simulink model "wlanhdlTimeAndFrequencySynchronization"  (R2025a)
settings: Solver=FixedStepDiscrete  StartTime=0.0  StopTime=stopTime  RelTol=1e-3
InitFcn:
  | wlanFrontEndInit;
values from neighbouring files (symbols this model uses):
  filterLatency = (wlanConfig.corrLen/filterUpsampleFactor)+filterUpsampleFactor+9    [wlanFrontEndInit.m]
  filterUpsampleFactor = 160e6/wlanConfig.Fs    [wlanFrontEndInit.m]
  Hd = dfilt.dffir(b)    [wlanFrontEndInit.m]
undefined symbols (not defined in the file or in its folder): Add, Shift, wlanConfig
libraries: simulink x14, hdlsllib x9, dspsrcs4 x3, dspsigops x3, dsphdlsigops2 x2, dsphdlmathfun2 x2, dsphdlfiltering2 x2
(part 1 of 2)
settings Model: DataTypeOverride=Off  Creator=The MathWorks, Inc.  LastModifiedBy=The MathWorks, Inc.
settings SolverCC: MaxZcPerStep=1.0
settings OptimizationCC: BlockReduction=off  ConditionallyExecuteInputs=off  DefaultParameterBehavior=Inlined  ReuseModelBlockBuffer=off
settings DebuggingCC: AlgebraicLoopMsg=error  SaveWithParameterizedLinksMsg=none  SingleTaskRateTransMsg=error  UnconnectedInputMsg=warning  UnconnectedOutputMsg=warning  UnconnectedLineMsg=warning
settings HardwareCC: ProdBitPerPointer=32.0  ProdBitPerSizeT=32.0  ProdBitPerPtrDiffT=32.0  ProdLargestAtomicFloat=None  ProdIntDivRoundTo=Undefined  ProdEndianess=Unspecified  ProdWordSize=32.0  ProdHWDeviceType=ASIC/FPGA->ASIC/FPGA  TargetBitPerPointer=64.0  TargetBitPerSizeT=64.0  TargetBitPerPtrDiffT=64.0  TargetLongLongMode=on  TargetIntDivRoundTo=Zero  TargetEndianess=LittleEndian  TargetWordSize=64.0  TargetHWDeviceType=Custom Processor->MATLAB Host Computer  ProdEqTarget=off
settings ModelReferenceCC: EnableRefExpFcnMdlSchedulingChecks=on
settings RTWCC: GPUComputeCapability=3.5  DLArmComputeVersion=19.05

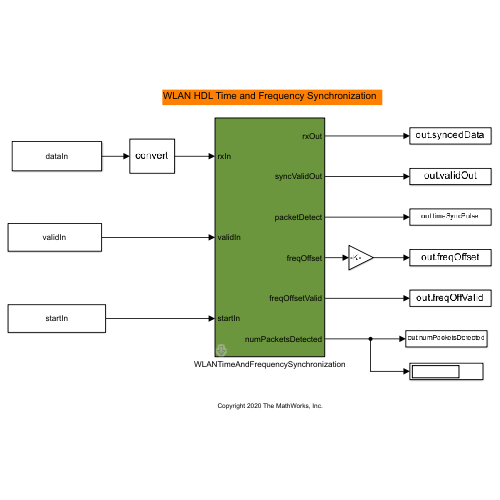
[thumbnail: Simulink's stored preview of the top-level diagram]
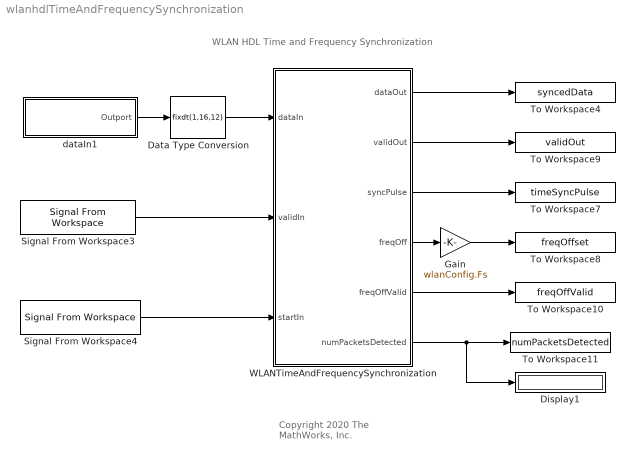
== system wlanhdlTimeAndFrequencySynchronization ==
  note: Copyright 2020 The MathWorks, Inc.
  note: WLAN HDL Time and Frequency Synchronization
  Data Type Conversion : DataTypeConversion  OutDataTypeStr=fixdt(1,16,12)  SaturateOnIntegerOverflow=off  RndMeth=Floor
  Display1 : Display
  Gain : Gain  Gain=wlanConfig.Fs
  Signal From Workspace3 : dspsrcs4/Signal From Workspace  X=validIn  Ts=1/wlanConfig.Fs  nsamps=1  OutputAfterFinalValue=Setting to zero  ignoreOrWarnInputAndFrameLengths=off  OutputFrames=off
  Signal From Workspace4 : dspsrcs4/Signal From Workspace  X=startIn  Ts=1/wlanConfig.Fs  nsamps=1  OutputAfterFinalValue=Setting to zero  ignoreOrWarnInputAndFrameLengths=off  OutputFrames=off
  To Workspace10 : ToWorkspace  VariableName=freqOffValid  SampleTime=-1
      settings: Save2DSignal=2-D array (concatenate along first dimension)
  To Workspace11 : ToWorkspace  VariableName=numPacketsDetected  SampleTime=-1
      settings: Save2DSignal=2-D array (concatenate along first dimension)
  To Workspace4 : ToWorkspace  VariableName=syncedData  SampleTime=-1
      settings: Save2DSignal=2-D array (concatenate along first dimension)
  To Workspace7 : ToWorkspace  VariableName=timeSyncPulse  SampleTime=-1
      settings: Save2DSignal=2-D array (concatenate along first dimension)
  To Workspace8 : ToWorkspace  VariableName=freqOffset  SampleTime=-1
      settings: Save2DSignal=2-D array (concatenate along first dimension)
  To Workspace9 : ToWorkspace  VariableName=validOut  SampleTime=-1
      settings: Save2DSignal=2-D array (concatenate along first dimension)
  WLANTimeAndFrequencySynchronization : Subsystem  mask(WLAN Front end application){chanBW=20MHz}
      mask prompts: chanBW "Channel bandwidth:"
      mask help: Performs time and frequency synchronization.
      mask Help: eval('showExample(''whdl/WLANHDLTimeAndFrequencySynchronizationExample'')')
      mask TypeOptions chanBW: 20MHz | 40MHz | 80MHz
      mask DialogControl DescGroupVar Prompt: WLAN Time and Frequency Synchronization
      mask DialogControl DescTextVar Prompt: Perform time and frequency synchronization.
      mask DialogControl ParameterGroupVar Prompt: Main
      mask Display:
      | port_label('input',1,'rxIn');
      | port_label('input',2,'validIn');
      | port_label('input',3,'startIn');
      | port_label('output',1,'rxOut');
      | port_label('output',2,'syncValidOut');
      | port_label('output',3,'packetDetect');
      | port_label('output',4,'freqOffset');
      | port_label('output',5,'freqOffsetValid');
      | 
      | port_label('output',6,'numPacketsDetected');
  dataIn1 : Subsystem
      mask Display: disp('dataIn');
  wires:
  Signal From Workspace3/1 -> WLANTimeAndFrequencySynchronization/2(validIn)
  WLANTimeAndFrequencySynchronization/5(freqOffValid) -> To Workspace10/1
  WLANTimeAndFrequencySynchronization/6(numPacketsDetected) -> To Workspace11/1, Display1/1
  WLANTimeAndFrequencySynchronization/3(syncPulse) -> To Workspace7/1
  Signal From Workspace4/1 -> WLANTimeAndFrequencySynchronization/3(startIn)
  WLANTimeAndFrequencySynchronization/2(validOut) -> To Workspace9/1
  WLANTimeAndFrequencySynchronization/1(dataOut) -> To Workspace4/1
  Data Type Conversion/1 -> WLANTimeAndFrequencySynchronization/1(dataIn)
  dataIn1/1(Outport) -> Data Type Conversion/1
  WLANTimeAndFrequencySynchronization/4(freqOff) -> Gain/1
  Gain/1 -> To Workspace8/1

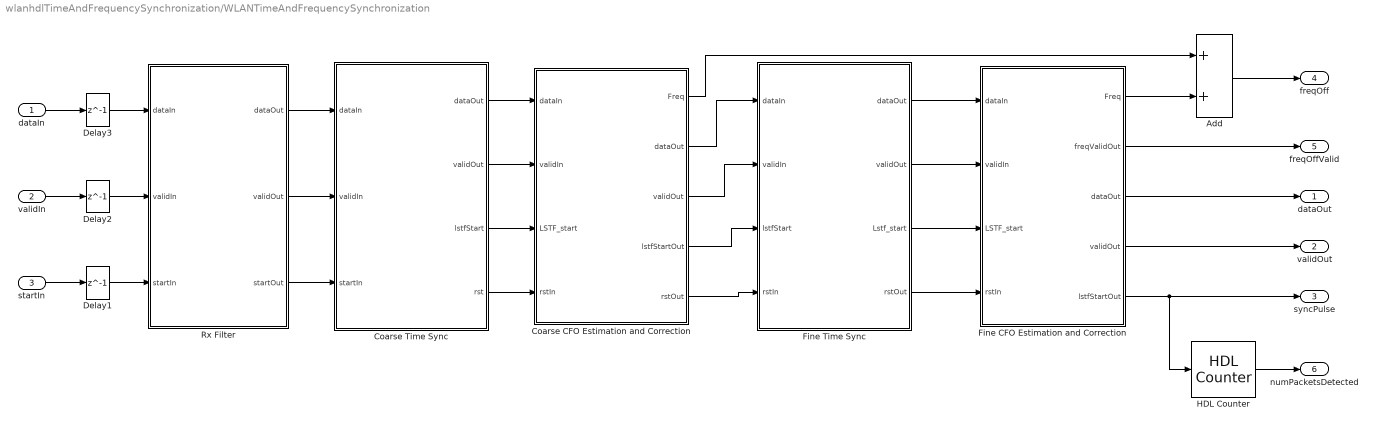
== system wlanhdlTimeAndFrequencySynchronization/WLANTimeAndFrequencySynchronization ==
  dataIn : Inport
  validIn : Inport  Port=2
  startIn : Inport  Port=3
  Add : Sum
  Coarse CFO Estimation and Correction : Subsystem
  Coarse Time Sync : Subsystem
  Delay1 : Delay  DelayLength=1  InitialCondition=0
  Delay2 : Delay  DelayLength=1  InitialCondition=0
  Delay3 : Delay  DelayLength=1  InitialCondition=0
  Fine CFO Estimation and Correction : Subsystem
  Fine Time Sync : Subsystem
  HDL Counter : hdlsllib/Sources/HDL Counter  CountType=Count limited  CountInit=0  CountStep=1  CountMax=65535  CountFromType=Initial value  CountFrom=0  CountResetPort=off  CountLoadPort=off  CountEnbPort=on  CountDirPort=off  CountHitOutputPort=off  CountDataType=Unsigned  CountWordLen=16  CountFracLen=0  CountSampTime=1
      link override Add_wrap/Compare To Constant/Compare: Operator=>  OutDataTypeStr=boolean
      link override Sub_wrap/Compare To Constant/Compare: Operator=<  OutDataTypeStr=boolean
      link override const_load_val: OutDataTypeStr=fixdt(issigned,CountWordLen,CountFracLen,'DataTypeOverride','Off')
  Rx Filter : Subsystem
  dataOut : Outport
  validOut : Outport  Port=2
  syncPulse : Outport  Port=3
  freqOff : Outport  Port=4
  freqOffValid : Outport  Port=5
  numPacketsDetected : Outport  Port=6
  wires:
  Add/1 -> freqOff/1
  validIn/1 -> Delay2/1
  dataIn/1 -> Delay3/1
  startIn/1 -> Delay1/1
  Delay1/1 -> Rx Filter/3(startIn)
  Rx Filter/3(startOut) -> Coarse Time Sync/3(startIn)
  Fine CFO Estimation and Correction/2(freqValidOut) -> freqOffValid/1
  HDL Counter/1 -> numPacketsDetected/1
  Delay3/1 -> Rx Filter/1(dataIn)
  Delay2/1 -> Rx Filter/2(validIn)
  Rx Filter/1(dataOut) -> Coarse Time Sync/1(dataIn)
  Rx Filter/2(validOut) -> Coarse Time Sync/2(validIn)
  Coarse Time Sync/1(dataOut) -> Coarse CFO Estimation and Correction/1(dataIn)
  Coarse Time Sync/2(validOut) -> Coarse CFO Estimation and Correction/2(validIn)
  Coarse Time Sync/3(lstfStart) -> Coarse CFO Estimation and Correction/3(LSTF_start)
  Coarse Time Sync/4(rst) -> Coarse CFO Estimation and Correction/4(rstIn)
  Coarse CFO Estimation and Correction/1(Freq) -> Add/1
  Coarse CFO Estimation and Correction/2(dataOut) -> Fine Time Sync/1(dataIn)
  Coarse CFO Estimation and Correction/3(validOut) -> Fine Time Sync/2(validIn)
  Coarse CFO Estimation and Correction/4(lstfStartOut) -> Fine Time Sync/3(lstfStart)
  Coarse CFO Estimation and Correction/5(rstOut) -> Fine Time Sync/4(rstIn)
  Fine CFO Estimation and Correction/5(lstfStartOut) -> syncPulse/1, HDL Counter/1
  Fine Time Sync/1(dataOut) -> Fine CFO Estimation and Correction/1(dataIn)
  Fine Time Sync/2(validOut) -> Fine CFO Estimation and Correction/2(validIn)
  Fine Time Sync/3(Lstf_start) -> Fine CFO Estimation and Correction/3(LSTF_start)
  Fine Time Sync/4(rstOut) -> Fine CFO Estimation and Correction/4(rstIn)
  Fine CFO Estimation and Correction/1(Freq) -> Add/2
  Fine CFO Estimation and Correction/3(dataOut) -> dataOut/1
  Fine CFO Estimation and Correction/4(validOut) -> validOut/1

== system wlanhdlTimeAndFrequencySynchronization/dataIn1 ==
  Signal From Workspace : dspsrcs4/Signal From Workspace  X=inputWaveform  Ts=1/wlanConfig.Fs  nsamps=1  OutputAfterFinalValue=Setting to zero  ignoreOrWarnInputAndFrameLengths=off  OutputFrames=off
  Outport : Outport
  wires:
  Signal From Workspace/1 -> Outport/1

== system wlanhdlTimeAndFrequencySynchronization/WLANTimeAndFrequencySynchronization/Coarse CFO Estimation and Correction ==
  dataIn : Inport
  validIn : Inport  Port=2
  LSTF_start : Inport  Port=3
  rstIn : Inport  Port=4
  Coarse CFO Correction : Subsystem
  Coarse CFO Estimation : Subsystem
  Freq : Outport
  dataOut : Outport  Port=2
  validOut : Outport  Port=3
  lstfStartOut : Outport  Port=4
  rstOut : Outport  Port=5
  wires:
  Coarse CFO Estimation/3(validData) -> Coarse CFO Correction/3(validIn)
  Coarse CFO Correction/3(validOut) -> validOut/1
  Coarse CFO Estimation/4(lstfStart) -> Coarse CFO Correction/4(lstfStartIn)
  Coarse CFO Estimation/1(Freq) -> Coarse CFO Correction/1(freq)
  LSTF_start/1 -> Coarse CFO Estimation/3(LSTF_start)
  validIn/1 -> Coarse CFO Estimation/2(validIn)
  Coarse CFO Estimation/5(rstOut) -> Coarse CFO Correction/5(rstIn)
  Coarse CFO Estimation/2(dataOut) -> Coarse CFO Correction/2(dataIn)
  dataIn/1 -> Coarse CFO Estimation/1(dataIn)
  Coarse CFO Correction/2(dataOut) -> dataOut/1
  rstIn/1 -> Coarse CFO Estimation/4(rstIn)
  Coarse CFO Correction/4(lstfStartOut) -> lstfStartOut/1
  Coarse CFO Correction/5(rstOut) -> rstOut/1
  Coarse CFO Correction/1(freqOut) -> Freq/1

== system wlanhdlTimeAndFrequencySynchronization/WLANTimeAndFrequencySynchronization/Coarse Time Sync ==
  dataIn : Inport
  validIn : Inport  Port=2
  startIn : Inport  Port=3
  Correlator : Subsystem
  Delay4 : Delay  DelayLength=7
  Delay6 : Delay  DelayLength=7
  Energy Calculator : Subsystem
  Peak Detector : Subsystem
  Stream Synchronizer : Subsystem
  dataOut : Outport  VectorParamsAs1DForOutWhenUnconnected=off
  validOut : Outport  Port=2  VectorParamsAs1DForOutWhenUnconnected=off
  lstfStart : Outport  Port=3  VectorParamsAs1DForOutWhenUnconnected=off
  rst : Outport  Port=4  VectorParamsAs1DForOutWhenUnconnected=off
  wires:
  startIn/1 -> rst/1, Correlator/3(startIn)
  Peak Detector/3(dataOut) -> dataOut/1
  validIn/1 -> Delay6/1, Correlator/2(validIn), Energy Calculator/4(validIn)
  Delay4/1 -> Stream Synchronizer/2(dataIn)
  Delay6/1 -> Stream Synchronizer/3(dataValid)
  Correlator/2(validOut) -> Energy Calculator/2(corrValidIn), Stream Synchronizer/1(corrValid)
  dataIn/1 -> Energy Calculator/3(dataIn), Delay4/1, Correlator/1(dataIn)
  Peak Detector/2(validOut) -> validOut/1
  Energy Calculator/2(energyOut) -> Peak Detector/2(energyIn)
  Energy Calculator/3(validOut) -> Peak Detector/3(corrValid)
  Peak Detector/1(lstfStart) -> lstfStart/1
  Correlator/1(dataOut) -> Energy Calculator/1(corrIn)
  Energy Calculator/1(corrOut) -> Peak Detector/1(corrIn)
  Stream Synchronizer/1(dataOut) -> Peak Detector/4(dataIn)
  Stream Synchronizer/2(validOut) -> Peak Detector/5(dataValid)

== system wlanhdlTimeAndFrequencySynchronization/WLANTimeAndFrequencySynchronization/Fine CFO Estimation and Correction ==
  dataIn : Inport
  validIn : Inport  Port=2
  LSTF_start : Inport  Port=3
  rstIn : Inport  Port=4
  Fine CFO Correction : Subsystem
  Fine CFO Estimation : Subsystem
  Freq : Outport
  freqValidOut : Outport  Port=2
  dataOut : Outport  Port=3
  validOut : Outport  Port=4
  lstfStartOut : Outport  Port=5
  wires:
  Fine CFO Estimation/4(validOut) -> Fine CFO Correction/4(validIn)
  Fine CFO Estimation/1(Freq) -> Fine CFO Correction/1(freqIn)
  validIn/1 -> Fine CFO Estimation/2(validIn)
  Fine CFO Estimation/5(lstfStart) -> Fine CFO Correction/5(lstfStartIn)
  Fine CFO Estimation/3(dataOut) -> Fine CFO Correction/3(dataIn)
  dataIn/1 -> Fine CFO Estimation/1(dataIn)
  Fine CFO Estimation/2(freqValidOut) -> Fine CFO Correction/2(freqValidIn)
  LSTF_start/1 -> Fine CFO Estimation/3(LSTF_start)
  rstIn/1 -> Fine CFO Estimation/4(rstIn)
  Fine CFO Correction/5(lstfStartOut) -> lstfStartOut/1
  Fine CFO Correction/4(validOut) -> validOut/1
  Fine CFO Correction/3(dataOut) -> dataOut/1
  Fine CFO Correction/1(freqOut) -> Freq/1
  Fine CFO Correction/2(freqValidOut) -> freqValidOut/1

== system wlanhdlTimeAndFrequencySynchronization/WLANTimeAndFrequencySynchronization/Fine Time Sync ==
  dataIn : Inport
  validIn : Inport  Port=2
  lstfStart : Inport  Port=3
  rstIn : Inport  Port=4
  Correlator : Subsystem
  Peak Searcher : Subsystem
  dataOut : Outport  VectorParamsAs1DForOutWhenUnconnected=off
  validOut : Outport  Port=2  VectorParamsAs1DForOutWhenUnconnected=off
  Lstf_start : Outport  Port=3  VectorParamsAs1DForOutWhenUnconnected=off
  rstOut : Outport  Port=4  VectorParamsAs1DForOutWhenUnconnected=off
  wires:
  validIn/1 -> Correlator/2(validIn)
  dataIn/1 -> Correlator/1(dataIn)
  lstfStart/1 -> Correlator/3(startIn)
  Correlator/1(corrOut) -> Peak Searcher/1(corrIn)
  Correlator/2(corrValid) -> Peak Searcher/2(corrValid)
  Correlator/3(startOut) -> Peak Searcher/3(startIn)
  Peak Searcher/1(lstfStart) -> Lstf_start/1
  Peak Searcher/2(validOut) -> validOut/1
  Peak Searcher/3(dataOut) -> dataOut/1
  Correlator/4(dataOut) -> Peak Searcher/4(dataIn)
  Correlator/5(validOut) -> Peak Searcher/5(validIn)
  rstIn/1 -> rstOut/1, Peak Searcher/6(rstIn), Correlator/4(rstIn)

== system wlanhdlTimeAndFrequencySynchronization/WLANTimeAndFrequencySynchronization/Rx Filter ==
  dataIn : Inport
  validIn : Inport  Port=2
  startIn : Inport  Port=3
  DTConverter : MATLAB Function  TreatAsAtomicUnit=on
  Delay : Delay  DelayLength=33
  Discrete FIR Filter : dsphdlfiltering2/Discrete FIR Filter  NumeratorSource=Property  Numerator=Hd.Numerator  NumeratorPrototype=[]  FilterStructure=Direct form systolic  SerializationOption=Minimum number of cycles between valid input samples  NumCycles=2  NumberOfMultipliers=2  SimulateUsing=Code generation  roundingMode=Floor  overflowMode=off  CoefficientsDataTypeStr=Inherit: Same word length as input  OutputDataTypeStr=Inherit: Same word length as input  ResetInputPort=on  HDLGlobalReset=off  CoeffMultiplier=Multiplier  UseMultForPow2Coeff=on  FrameInputSymmOptim=off
  dataOut : Outport
  validOut : Outport  Port=2
  startOut : Outport  Port=3
  wires:
  dataIn/1 -> DTConverter/1(dataIn1), Discrete FIR Filter/1
  validIn/1 -> Discrete FIR Filter/2
  Discrete FIR Filter/2 -> validOut/1
  Discrete FIR Filter/1 -> DTConverter/2(dataIn2)
  DTConverter/1(dataOut) -> dataOut/1
  startIn/1 -> Discrete FIR Filter/3, Delay/1
  Delay/1 -> startOut/1

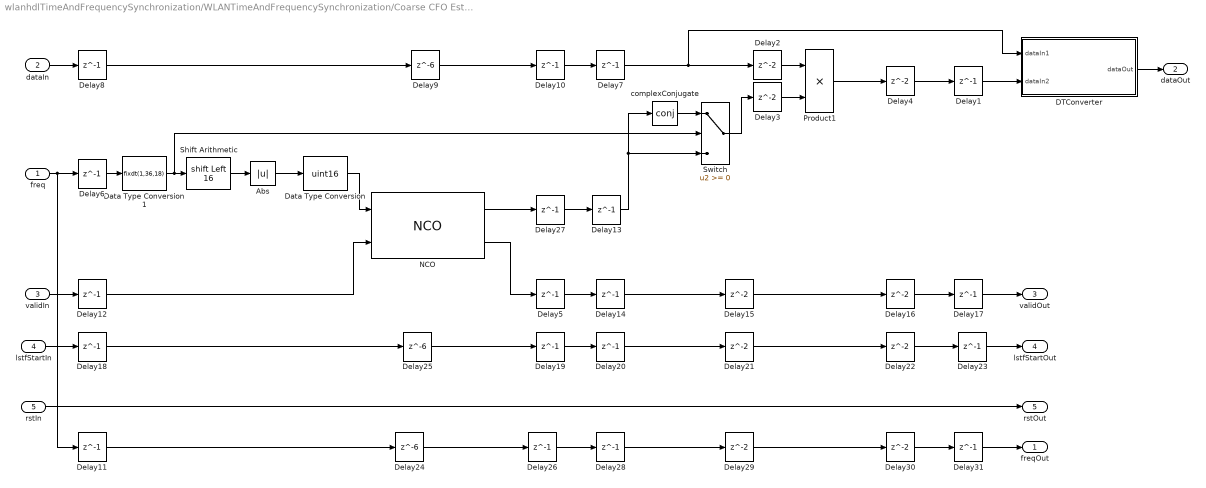
== system wlanhdlTimeAndFrequencySynchronization/WLANTimeAndFrequencySynchronization/Coarse CFO Estimation and Correction/Coarse CFO Correction ==
  freq : Inport
  dataIn : Inport  Port=2
  validIn : Inport  Port=3
  lstfStartIn : Inport  Port=4
  rstIn : Inport  Port=5
  Abs : Abs  SaturateOnIntegerOverflow=off
  DTConverter : MATLAB Function  TreatAsAtomicUnit=on
  Data Type Conversion : DataTypeConversion  OutDataTypeStr=uint16  RndMeth=Round  SaturateOnIntegerOverflow=off
  Data Type Conversion1 : DataTypeConversion  OutDataTypeStr=fixdt(1,36,18)  SaturateOnIntegerOverflow=off  RndMeth=Floor
  Delay{1,5..8,10..14,17..20,23,26..28,31} (19 alike) : Delay  DelayLength=1  InitialCondition=0  UseCircularBuffer=on
  Delay{2..4,15..16,21..22,29..30} (9 alike) : Delay  InitialCondition=0  UseCircularBuffer=on
  Delay24 : Delay  DelayLength=6  InitialCondition=0  UseCircularBuffer=on
  Delay25 : Delay  DelayLength=6  InitialCondition=0  UseCircularBuffer=on
  Delay9 : Delay  DelayLength=6  InitialCondition=0  UseCircularBuffer=on
  NCO : dsphdlsigops2/NCO  PhaseIncrementSource=Input port  PhaseIncrement=100  PhaseOffsetSource=Property  PhaseOffset=0  DitherSource=None  NumDitherBits=4  SamplesPerFrame=1  LUTCompress=off  ResetAction=off  Waveform=Complex exponential  PhasePort=off  SimulateUsing=Code generation  AccumulatorWL=16  PhaseQuantization=on  NumQuantizerAccumulatorBits=16  OutputDataType=Binary point scaling  OutputWL=16  OutputFL=14
  Product1 : Product
  Shift Arithmetic : ArithShift  BitShiftNumber=16  BitShiftDirection=Left
  Switch : Switch  SaturateOnIntegerOverflow=off  InputSameDT=off
  complexConjugate : Math  Operator=conj  SignedPower=on
  freqOut : Outport  VectorParamsAs1DForOutWhenUnconnected=off
  dataOut : Outport  Port=2  VectorParamsAs1DForOutWhenUnconnected=off
  validOut : Outport  Port=3  VectorParamsAs1DForOutWhenUnconnected=off
  lstfStartOut : Outport  Port=4  VectorParamsAs1DForOutWhenUnconnected=off
  rstOut : Outport  Port=5  VectorParamsAs1DForOutWhenUnconnected=off
  wires:
  Delay25/1 -> Delay19/1
  NCO/2 -> Delay5/1
  Delay9/1 -> Delay10/1
  Delay23/1 -> lstfStartOut/1
  Delay22/1 -> Delay23/1
  Delay21/1 -> Delay22/1
  Delay20/1 -> Delay21/1
  Delay19/1 -> Delay20/1
  Delay18/1 -> Delay25/1
  lstfStartIn/1 -> Delay18/1
  Delay5/1 -> Delay14/1
  freq/1 -> Delay11/1, Delay6/1
  Delay4/1 -> Delay1/1
  dataIn/1 -> Delay8/1
  Delay17/1 -> validOut/1
  Delay3/1 -> Product1/2
  Delay16/1 -> Delay17/1
  validIn/1 -> Delay12/1
  Delay10/1 -> Delay7/1
  Delay15/1 -> Delay16/1
  Delay2/1 -> Product1/1
  Product1/1 -> Delay4/1
  Delay13/1 -> complexConjugate/1, Switch/3
  Delay8/1 -> Delay9/1
  Delay7/1 -> DTConverter/1(dataIn1), Delay2/1
  Delay14/1 -> Delay15/1
  Delay27/1 -> Delay13/1
  Data Type Conversion/1 -> NCO/1
  Delay12/1 -> NCO/2
  NCO/1 -> Delay27/1
  rstIn/1 -> rstOut/1
  Delay6/1 -> Data Type Conversion1/1
  Data Type Conversion1/1 -> Switch/2, Shift Arithmetic/1
  DTConverter/1(dataOut) -> dataOut/1
  Delay1/1 -> DTConverter/2(dataIn2)
  complexConjugate/1 -> Switch/1
  Switch/1 -> Delay3/1
  Shift Arithmetic/1 -> Abs/1
  Abs/1 -> Data Type Conversion/1
  Delay11/1 -> Delay24/1
  Delay24/1 -> Delay26/1
  Delay26/1 -> Delay28/1
  Delay28/1 -> Delay29/1
  Delay29/1 -> Delay30/1
  Delay30/1 -> Delay31/1
  Delay31/1 -> freqOut/1

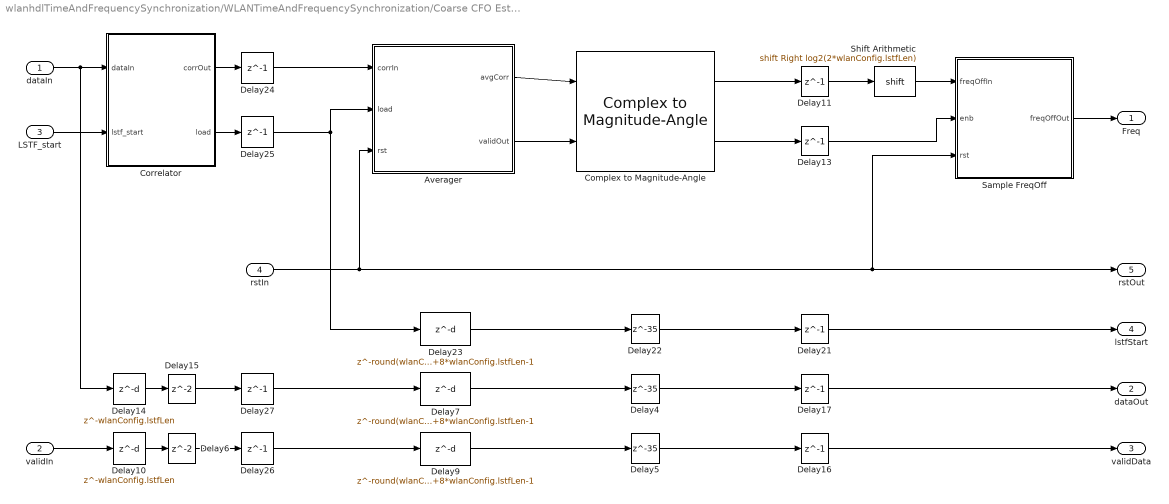
== system wlanhdlTimeAndFrequencySynchronization/WLANTimeAndFrequencySynchronization/Coarse CFO Estimation and Correction/Coarse CFO Estimation ==
  dataIn : Inport
  validIn : Inport  Port=2
  LSTF_start : Inport  Port=3
  rstIn : Inport  Port=4
  Averager : Subsystem
  Complex to Magnitude-Angle : dsphdlmathfun2/Complex to Magnitude-Angle  NumIterationsSource=Auto  NumIterations=30  OutputFormat=Angle  AngleFormat=Normalized  ScaleOutput=off  ScalingMethod=Shift-Add  SimulateUsing=Code generation
  Correlator : Subsystem
  Delay10 : Delay  DelayLength=wlanConfig.lstfLen  InitialCondition=0
  Delay{11,13,16..17,21} (5 alike) : Delay  DelayLength=1  InitialCondition=0  UseCircularBuffer=on
  Delay14 : Delay  DelayLength=wlanConfig.lstfLen  InitialCondition=0
  Delay15 : Delay  InitialCondition=0  UseCircularBuffer=on
  Delay22 : Delay  DelayLength=35  InitialCondition=0  UseCircularBuffer=on
  Delay23 : Delay  DelayLength=round(wlanConfig.lstfLen*0.75)+8*wlanConfig.lstfLen-1  InitialCondition=0  UseCircularBuffer=on
  Delay{24..27} (4 alike) : Delay  DelayLength=1
  Delay4 : Delay  DelayLength=35  InitialCondition=0  UseCircularBuffer=on
  Delay5 : Delay  DelayLength=35  InitialCondition=0  UseCircularBuffer=on
  Delay6 : Delay  InitialCondition=0  UseCircularBuffer=on
  Delay7 : Delay  DelayLength=round(wlanConfig.lstfLen*0.75)+8*wlanConfig.lstfLen-1  InitialCondition=0  UseCircularBuffer=on
  Delay9 : Delay  DelayLength=round(wlanConfig.lstfLen*0.75)+8*wlanConfig.lstfLen-1  InitialCondition=0  UseCircularBuffer=on
  Sample FreqOff : MATLAB Function  TreatAsAtomicUnit=on
  Shift Arithmetic : ArithShift  BitShiftNumber=log2(2*wlanConfig.lstfLen)  BitShiftDirection=Right
  Freq : Outport  VectorParamsAs1DForOutWhenUnconnected=off
  dataOut : Outport  Port=2  VectorParamsAs1DForOutWhenUnconnected=off
  validData : Outport  Port=3  VectorParamsAs1DForOutWhenUnconnected=off
  lstfStart : Outport  Port=4  VectorParamsAs1DForOutWhenUnconnected=off
  rstOut : Outport  Port=5  VectorParamsAs1DForOutWhenUnconnected=off
  wires:
  validIn/1 -> Delay10/1
  dataIn/1 -> Delay14/1, Correlator/1(dataIn)
  LSTF_start/1 -> Correlator/2(lstf_start)
  Delay9/1 -> Delay5/1
  Complex to Magnitude-Angle/2 -> Delay13/1
  Delay5/1 -> Delay16/1
  Delay4/1 -> Delay17/1
  Complex to Magnitude-Angle/1 -> Delay11/1
  Delay16/1 -> validData/1
  Delay17/1 -> dataOut/1
  Delay10/1 -> Delay6/1
  Delay6/1 -> Delay26/1
  Delay11/1 -> Shift Arithmetic/1
  Delay7/1 -> Delay4/1
  Delay26/1 -> Delay9/1
  Delay14/1 -> Delay15/1
  Delay15/1 -> Delay27/1
  Delay27/1 -> Delay7/1
  Delay22/1 -> Delay21/1
  Correlator/2(load) -> Delay25/1
  Delay23/1 -> Delay22/1
  Delay21/1 -> lstfStart/1
  Delay25/1 -> Delay23/1, Averager/2(load)
  Shift Arithmetic/1 -> Sample FreqOff/1(freqOffIn)
  Sample FreqOff/1(freqOffOut) -> Freq/1
  Delay13/1 -> Sample FreqOff/2(enb)
  rstIn/1 -> rstOut/1, Sample FreqOff/3(rst), Averager/3(rst)
  Correlator/1(corrOut) -> Delay24/1
  Averager/1(avgCorr) -> Complex to Magnitude-Angle/1
  Averager/2(validOut) -> Complex to Magnitude-Angle/2
  Delay24/1 -> Averager/1(corrIn)

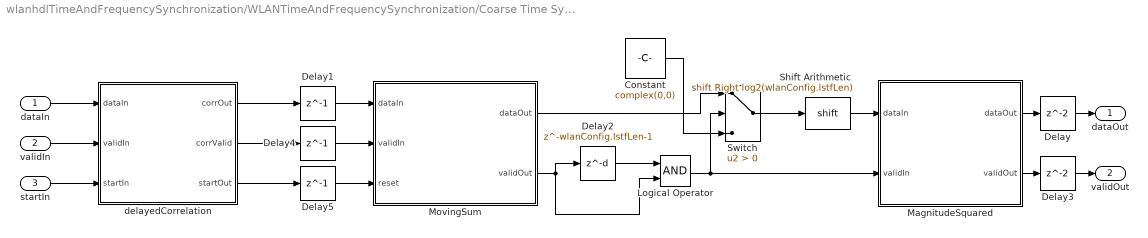
== system wlanhdlTimeAndFrequencySynchronization/WLANTimeAndFrequencySynchronization/Coarse Time Sync/Correlator ==
  dataIn : Inport
  validIn : Inport  Port=2
  startIn : Inport  Port=3
  Constant : Constant  Value=complex(0,0)  VectorParams1D=off  OutDataTypeStr=Inherit: Inherit via back propagation  SampleTime=-1
  Delay : Delay
  Delay1 : Delay  DelayLength=1
  Delay2 : Delay  DelayLength=wlanConfig.lstfLen-1
  Delay3 : Delay
  Delay4 : Delay  DelayLength=1
  Delay5 : Delay  DelayLength=1
  Logical Operator : Logic  AllPortsSameDT=off  OutDataTypeStr=boolean
  MagnitudeSquared : Subsystem
  MovingSum : Subsystem  InitFcn=Simulink.suppressDiagnostic(gcb, 'SimulinkFixedPoint:util:Overflowoccurred');
  Shift Arithmetic : ArithShift  BitShiftNumber=log2(wlanConfig.lstfLen)  BitShiftDirection=Right
  Switch : Switch  Criteria=u2 > Threshold  SaturateOnIntegerOverflow=off  InputSameDT=off
  delayedCorrelation : Subsystem
  dataOut : Outport
  validOut : Outport  Port=2
  wires:
  MagnitudeSquared/2(validOut) -> Delay3/1
  MovingSum/2(validOut) -> Delay2/1, Logical Operator/2
  Switch/1 -> Shift Arithmetic/1
  Constant/1 -> Switch/3
  MovingSum/1(dataOut) -> Switch/1
  Logical Operator/1 -> MagnitudeSquared/2(validIn), Switch/2
  Delay2/1 -> Logical Operator/1
  MagnitudeSquared/1(dataOut) -> Delay/1
  Shift Arithmetic/1 -> MagnitudeSquared/1(dataIn)
  Delay/1 -> dataOut/1
  Delay3/1 -> validOut/1
  dataIn/1 -> delayedCorrelation/1(dataIn)
  validIn/1 -> delayedCorrelation/2(validIn)
  startIn/1 -> delayedCorrelation/3(startIn)
  delayedCorrelation/1(corrOut) -> Delay1/1
  delayedCorrelation/2(corrValid) -> Delay4/1
  delayedCorrelation/3(startOut) -> Delay5/1
  Delay1/1 -> MovingSum/1(dataIn)
  Delay4/1 -> MovingSum/2(validIn)
  Delay5/1 -> MovingSum/3(reset)

== system wlanhdlTimeAndFrequencySynchronization/WLANTimeAndFrequencySynchronization/Coarse Time Sync/Energy Calculator ==
  corrIn : Inport
  corrValidIn : Inport  Port=2
  dataIn : Inport  Port=3
  validIn : Inport  Port=4
  Delay : Delay  DelayLength=3
  magnitudeSquared : Subsystem
  streamSynchronizer : Subsystem
  corrOut : Outport
  energyOut : Outport  Port=2
  validOut : Outport  Port=3
  wires:
  validIn/1 -> magnitudeSquared/2(validIn)
  streamSynchronizer/1(dataOut) -> energyOut/1
  magnitudeSquared/1(energy) -> streamSynchronizer/2(energy)
  corrValidIn/1 -> streamSynchronizer/1(corrValid)
  streamSynchronizer/2(validOut) -> validOut/1
  magnitudeSquared/2(push) -> streamSynchronizer/3(dataValid)
  dataIn/1 -> magnitudeSquared/1(dataIn)
  corrIn/1 -> Delay/1
  Delay/1 -> corrOut/1

== system wlanhdlTimeAndFrequencySynchronization/WLANTimeAndFrequencySynchronization/Coarse Time Sync/Peak Detector ==
  note: Searching peak in LSTF region
  corrIn : Inport
  energyIn : Inport  Port=2
  corrValid : Inport  Port=3
  dataIn : Inport  Port=4
  dataValid : Inport  Port=5
  Delay1 : Delay  DelayLength=wlanConfig.lstfLen*10  InitialCondition=0  UseCircularBuffer=on
  Delay2 : Delay  DelayLength=wlanConfig.lstfLen*10  InitialCondition=0  UseCircularBuffer=on
  Logical Operator3 : Logic  AllPortsSameDT=off  OutDataTypeStr=boolean
  MATLAB Function1 : MATLAB Function  TreatAsAtomicUnit=on
  Relational Operator : RelationalOperator  Operator=>  OutDataTypeStr=boolean  InputSameDT=off
  considerFirstPeak : Subsystem
  searchStartOfFrame : MATLAB Function  TreatAsAtomicUnit=on
  lstfStart : Outport
  validOut : Outport  Port=2
  dataOut : Outport  Port=3
  wires:
  Relational Operator/1 -> searchStartOfFrame/1(thresholdValid)
  Logical Operator3/1 -> validOut/1, MATLAB Function1/1(syncEn)
  energyIn/1 -> Relational Operator/2
  dataValid/1 -> Delay1/1
  corrValid/1 -> searchStartOfFrame/2(valid)
  dataIn/1 -> Delay2/1
  Delay2/1 -> MATLAB Function1/2(dataIn)
  Delay1/1 -> MATLAB Function1/3(validIn), Logical Operator3/2
  MATLAB Function1/1(dataOut) -> dataOut/1
  searchStartOfFrame/1(syncOut) -> considerFirstPeak/1(peakIn)
  considerFirstPeak/1(peakOut) -> lstfStart/1
  considerFirstPeak/2(validOut) -> Logical Operator3/1
  corrIn/1 -> Relational Operator/1

== system wlanhdlTimeAndFrequencySynchronization/WLANTimeAndFrequencySynchronization/Coarse Time Sync/Stream Synchronizer ==
  corrValid : Inport
  dataIn : Inport  Port=2
  dataValid : Inport  Port=3
  Delay{1..4,6} (5 alike) : Delay  DelayLength=1
  Delay5 : Delay  DelayLength=wlanConfig.lstfLen-1
  Logical Operator8 : Logic  Operator=OR  AllPortsSameDT=off  OutDataTypeStr=boolean
  StreamSyncronizer : MATLAB Function  InitFcn=Simulink.suppressDiagnostic(gcb, 'Stateflow:Runtime:DataOverflowErrorMSLD');  TreatAsAtomicUnit=on  mask{depth=256}
      mask help: Synchronize two data streams with a FIFO.
  dataOut : Outport
  validOut : Outport  Port=2
  wires:
  dataIn/1 -> Delay4/1
  Delay6/1 -> StreamSyncronizer/3(push)
  Delay4/1 -> StreamSyncronizer/2(dataIn)
  StreamSyncronizer/2(validOut) -> Delay3/1
  dataValid/1 -> Delay6/1
  StreamSyncronizer/1(dataOut) -> Delay2/1
  Delay1/1 -> StreamSyncronizer/1(pop)
  Delay2/1 -> dataOut/1
  Delay3/1 -> validOut/1
  corrValid/1 -> Logical Operator8/2, Delay5/1
  Delay5/1 -> Logical Operator8/1
  Logical Operator8/1 -> Delay1/1

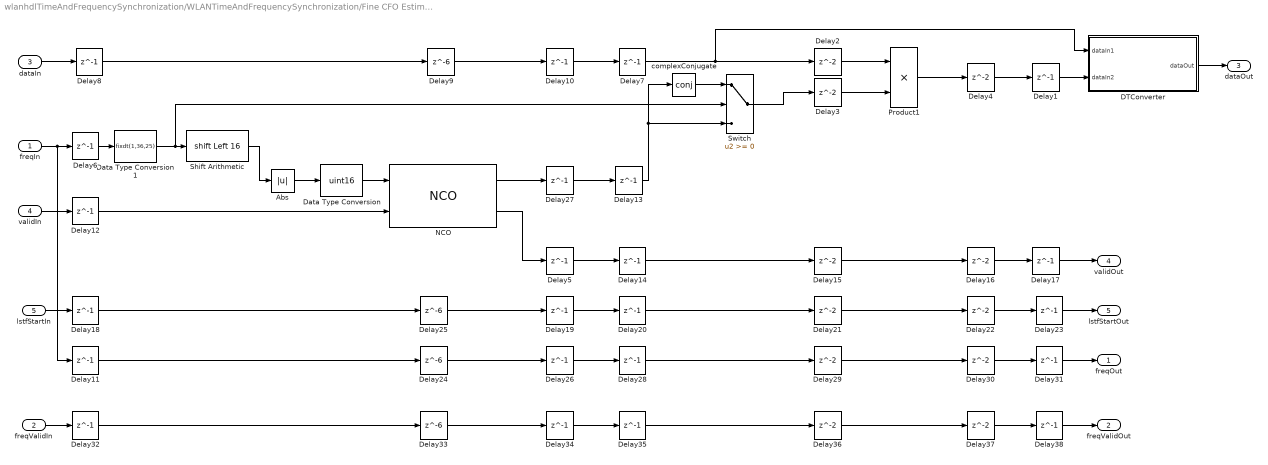
== system wlanhdlTimeAndFrequencySynchronization/WLANTimeAndFrequencySynchronization/Fine CFO Estimation and Correction/Fine CFO Correction ==
  freqIn : Inport
  freqValidIn : Inport  Port=2
  dataIn : Inport  Port=3
  validIn : Inport  Port=4
  lstfStartIn : Inport  Port=5
  Abs : Abs  SaturateOnIntegerOverflow=off
  DTConverter : MATLAB Function  TreatAsAtomicUnit=on
  Data Type Conversion : DataTypeConversion  OutDataTypeStr=uint16  RndMeth=Round  SaturateOnIntegerOverflow=off
  Data Type Conversion1 : DataTypeConversion  OutDataTypeStr=fixdt(1,36,25)  SaturateOnIntegerOverflow=off  RndMeth=Floor
  Delay{1,5..8,10..14,17..20,23,26..28,31..32,34..35,38} (23 alike) : Delay  DelayLength=1  InitialCondition=0  UseCircularBuffer=on
  Delay{2..4,15..16,21..22,29..30,36..37} (11 alike) : Delay  InitialCondition=0  UseCircularBuffer=on
  Delay{9,24..25,33} (4 alike) : Delay  DelayLength=6  InitialCondition=0  UseCircularBuffer=on
  NCO : dsphdlsigops2/NCO  PhaseIncrementSource=Input port  PhaseIncrement=100  PhaseOffsetSource=Property  PhaseOffset=0  DitherSource=None  NumDitherBits=4  SamplesPerFrame=1  LUTCompress=off  ResetAction=off  Waveform=Complex exponential  PhasePort=off  SimulateUsing=Code generation  AccumulatorWL=16  PhaseQuantization=on  NumQuantizerAccumulatorBits=16  OutputDataType=Binary point scaling  OutputWL=16  OutputFL=14
  Product1 : Product
  Shift Arithmetic : ArithShift  BitShiftNumber=16  BitShiftDirection=Left
  Switch : Switch  SaturateOnIntegerOverflow=off  InputSameDT=off
  complexConjugate : Math  Operator=conj  SignedPower=on
  freqOut : Outport  VectorParamsAs1DForOutWhenUnconnected=off
  freqValidOut : Outport  Port=2  VectorParamsAs1DForOutWhenUnconnected=off
  dataOut : Outport  Port=3  VectorParamsAs1DForOutWhenUnconnected=off
  validOut : Outport  Port=4  VectorParamsAs1DForOutWhenUnconnected=off
  lstfStartOut : Outport  Port=5  VectorParamsAs1DForOutWhenUnconnected=off
  wires:
  Delay25/1 -> Delay19/1
  NCO/2 -> Delay5/1
  Delay9/1 -> Delay10/1
  Delay23/1 -> lstfStartOut/1
  Delay22/1 -> Delay23/1
  Delay21/1 -> Delay22/1
  Delay20/1 -> Delay21/1
  Delay19/1 -> Delay20/1
  Delay18/1 -> Delay25/1
  lstfStartIn/1 -> Delay18/1
  Delay5/1 -> Delay14/1
  freqIn/1 -> Delay11/1, Delay6/1
  Delay4/1 -> Delay1/1
  dataIn/1 -> Delay8/1
  Delay17/1 -> validOut/1
  Delay3/1 -> Product1/2
  Delay16/1 -> Delay17/1
  validIn/1 -> Delay12/1
  Delay10/1 -> Delay7/1
  Delay15/1 -> Delay16/1
  Delay2/1 -> Product1/1
  Product1/1 -> Delay4/1
  Delay13/1 -> Switch/3, complexConjugate/1
  Delay8/1 -> Delay9/1
  Delay7/1 -> DTConverter/1(dataIn1), Delay2/1
  Delay14/1 -> Delay15/1
  Delay27/1 -> Delay13/1
  Data Type Conversion/1 -> NCO/1
  Delay12/1 -> NCO/2
  NCO/1 -> Delay27/1
  Delay6/1 -> Data Type Conversion1/1
  Data Type Conversion1/1 -> Switch/2, Shift Arithmetic/1
  DTConverter/1(dataOut) -> dataOut/1
  Delay1/1 -> DTConverter/2(dataIn2)
  Switch/1 -> Delay3/1
  complexConjugate/1 -> Switch/1
  Abs/1 -> Data Type Conversion/1
  Shift Arithmetic/1 -> Abs/1
  Delay11/1 -> Delay24/1
  Delay24/1 -> Delay26/1
  Delay26/1 -> Delay28/1
  Delay28/1 -> Delay29/1
  Delay29/1 -> Delay30/1
  Delay30/1 -> Delay31/1
  Delay31/1 -> freqOut/1
  freqValidIn/1 -> Delay32/1
  Delay32/1 -> Delay33/1
  Delay33/1 -> Delay34/1
  Delay34/1 -> Delay35/1
  Delay35/1 -> Delay36/1
  Delay36/1 -> Delay37/1
  Delay37/1 -> Delay38/1
  Delay38/1 -> freqValidOut/1

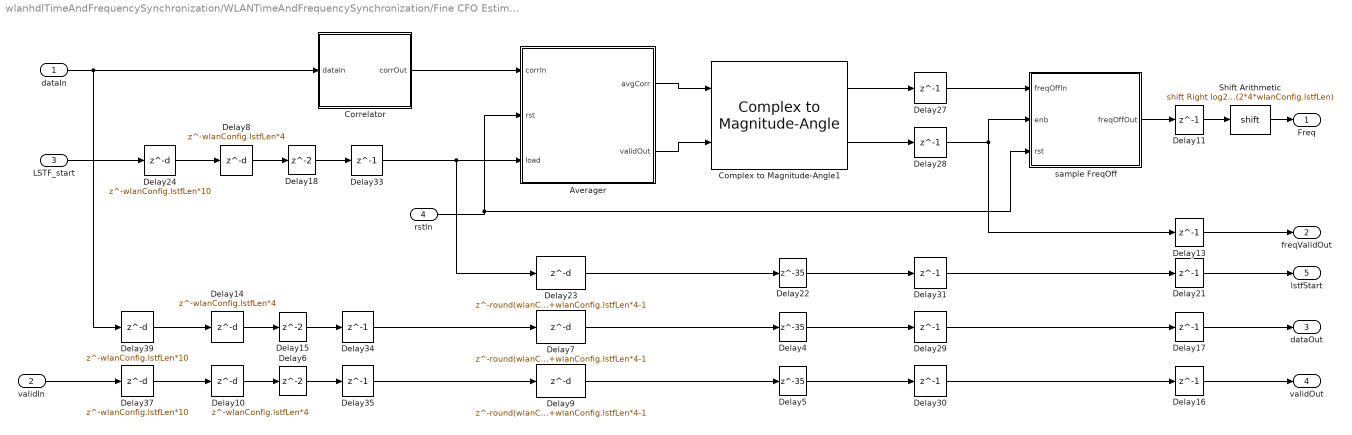
== system wlanhdlTimeAndFrequencySynchronization/WLANTimeAndFrequencySynchronization/Fine CFO Estimation and Correction/Fine CFO Estimation ==
  dataIn : Inport
  validIn : Inport  Port=2
  LSTF_start : Inport  Port=3
  rstIn : Inport  Port=4
  Averager : Subsystem
  Complex to Magnitude-Angle1 : dsphdlmathfun2/Complex to Magnitude-Angle  NumIterationsSource=Auto  NumIterations=30  OutputFormat=Angle  AngleFormat=Normalized  ScaleOutput=off  ScalingMethod=Shift-Add  SimulateUsing=Code generation
  Correlator : Subsystem
  Delay10 : Delay  DelayLength=wlanConfig.lstfLen*4  InitialCondition=0
  Delay{11,13,16..17,21} (5 alike) : Delay  DelayLength=1  InitialCondition=0  UseCircularBuffer=on
  Delay14 : Delay  DelayLength=wlanConfig.lstfLen*4  InitialCondition=0
  Delay15 : Delay  InitialCondition=0  UseCircularBuffer=on
  Delay18 : Delay  InitialCondition=0  UseCircularBuffer=on
  Delay22 : Delay  DelayLength=35  InitialCondition=0  UseCircularBuffer=on
  Delay23 : Delay  DelayLength=round(wlanConfig.lstfLen*2*0.75)+wlanConfig.lstfLen*4-1  InitialCondition=0  UseCircularBuffer=on
  Delay24 : Delay  DelayLength=wlanConfig.lstfLen*10  InitialCondition=0
  Delay{27..31,33..35} (8 alike) : Delay  DelayLength=1
  Delay37 : Delay  DelayLength=wlanConfig.lstfLen*10  InitialCondition=0
  Delay39 : Delay  DelayLength=wlanConfig.lstfLen*10  InitialCondition=0
  Delay4 : Delay  DelayLength=35  InitialCondition=0  UseCircularBuffer=on
  Delay5 : Delay  DelayLength=35  InitialCondition=0  UseCircularBuffer=on
  Delay6 : Delay  InitialCondition=0  UseCircularBuffer=on
  Delay7 : Delay  DelayLength=round(wlanConfig.lstfLen*2*0.75)+wlanConfig.lstfLen*4-1  InitialCondition=0  UseCircularBuffer=on
  Delay8 : Delay  DelayLength=wlanConfig.lstfLen*4  InitialCondition=0
  Delay9 : Delay  DelayLength=round(wlanConfig.lstfLen*2*0.75)+wlanConfig.lstfLen*4-1  InitialCondition=0  UseCircularBuffer=on
  Shift Arithmetic : ArithShift  BitShiftNumber=log2(2*4*wlanConfig.lstfLen)  BitShiftDirection=Right
  sample FreqOff : MATLAB Function  TreatAsAtomicUnit=on
  Freq : Outport  VectorParamsAs1DForOutWhenUnconnected=off
  freqValidOut : Outport  Port=2  VectorParamsAs1DForOutWhenUnconnected=off
  dataOut : Outport  Port=3  VectorParamsAs1DForOutWhenUnconnected=off
  validOut : Outport  Port=4  VectorParamsAs1DForOutWhenUnconnected=off
  lstfStart : Outport  Port=5  VectorParamsAs1DForOutWhenUnconnected=off
  wires:
  Delay9/1 -> Delay5/1
  Complex to Magnitude-Angle1/2 -> Delay28/1
  Complex to Magnitude-Angle1/1 -> Delay27/1
  Delay5/1 -> Delay30/1
  Delay4/1 -> Delay29/1
  sample FreqOff/1(freqOffOut) -> Delay11/1
  Delay13/1 -> freqValidOut/1
  Delay16/1 -> validOut/1
  Delay17/1 -> dataOut/1
  Delay10/1 -> Delay6/1
  Delay8/1 -> Delay18/1
  Delay6/1 -> Delay35/1
  Delay11/1 -> Shift Arithmetic/1
  Shift Arithmetic/1 -> Freq/1
  Delay7/1 -> Delay4/1
  Delay35/1 -> Delay9/1
  Delay14/1 -> Delay15/1
  Delay15/1 -> Delay34/1
  Delay34/1 -> Delay7/1
  Delay22/1 -> Delay31/1
  Delay23/1 -> Delay22/1
  Delay21/1 -> lstfStart/1
  Delay33/1 -> Averager/3(load), Delay23/1
  Delay24/1 -> Delay8/1
  LSTF_start/1 -> Delay24/1
  Delay18/1 -> Delay33/1
  Delay27/1 -> sample FreqOff/1(freqOffIn)
  Delay28/1 -> sample FreqOff/2(enb), Delay13/1
  Delay29/1 -> Delay17/1
  Delay30/1 -> Delay16/1
  Delay31/1 -> Delay21/1
  Delay37/1 -> Delay10/1
  Delay39/1 -> Delay14/1
  validIn/1 -> Delay37/1
  rstIn/1 -> sample FreqOff/3(rst), Averager/2(rst)
  dataIn/1 -> Correlator/1(dataIn), Delay39/1
  Correlator/1(corrOut) -> Averager/1(corrIn)
  Averager/1(avgCorr) -> Complex to Magnitude-Angle1/1
  Averager/2(validOut) -> Complex to Magnitude-Angle1/2

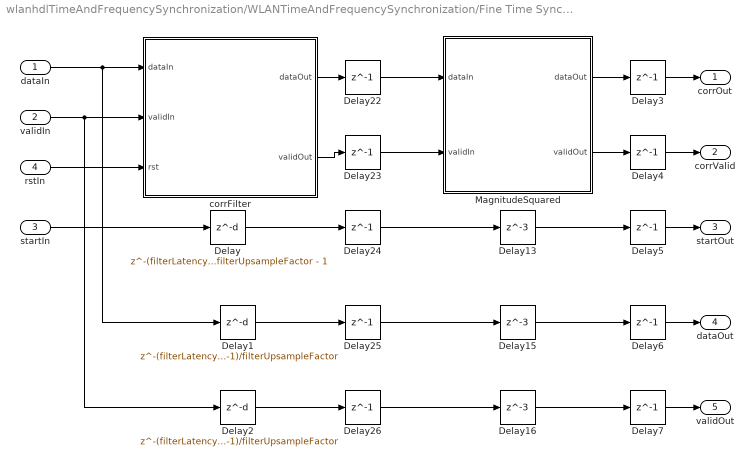
== system wlanhdlTimeAndFrequencySynchronization/WLANTimeAndFrequencySynchronization/Fine Time Sync/Correlator ==
  dataIn : Inport
  validIn : Inport  Port=2
  startIn : Inport  Port=3
  rstIn : Inport  Port=4
  Delay : Delay  DelayLength=(filterLatency+filterUpsampleFactor-1)/filterUpsampleFactor - 1
  Delay1 : Delay  DelayLength=(filterLatency+filterUpsampleFactor-1)/filterUpsampleFactor
  Delay13 : Delay  DelayLength=3
  Delay15 : Delay  DelayLength=3
  Delay16 : Delay  DelayLength=3
  Delay2 : Delay  DelayLength=(filterLatency+filterUpsampleFactor-1)/filterUpsampleFactor
  Delay{3..7,22..26} (10 alike) : Delay  DelayLength=1
  MagnitudeSquared : Subsystem
  corrFilter : Subsystem
  corrOut : Outport
  corrValid : Outport  Port=2
  startOut : Outport  Port=3
  dataOut : Outport  Port=4
  validOut : Outport  Port=5
  wires:
  corrFilter/1(dataOut) -> Delay22/1
  Delay13/1 -> Delay5/1
  startIn/1 -> Delay/1
  Delay22/1 -> MagnitudeSquared/1(dataIn)
  Delay24/1 -> Delay13/1
  Delay/1 -> Delay24/1
  Delay23/1 -> MagnitudeSquared/2(validIn)
  MagnitudeSquared/1(dataOut) -> Delay3/1
  corrFilter/2(validOut) -> Delay23/1
  MagnitudeSquared/2(validOut) -> Delay4/1
  Delay15/1 -> Delay6/1
  Delay16/1 -> Delay7/1
  validIn/1 -> Delay2/1, corrFilter/2(validIn)
  dataIn/1 -> corrFilter/1(dataIn), Delay1/1
  Delay1/1 -> Delay25/1
  Delay2/1 -> Delay26/1
  Delay26/1 -> Delay16/1
  Delay25/1 -> Delay15/1
  rstIn/1 -> corrFilter/3(rst)
  Delay3/1 -> corrOut/1
  Delay4/1 -> corrValid/1
  Delay5/1 -> startOut/1
  Delay6/1 -> dataOut/1
  Delay7/1 -> validOut/1

== system wlanhdlTimeAndFrequencySynchronization/WLANTimeAndFrequencySynchronization/Fine Time Sync/Peak Searcher ==
  corrIn : Inport
  corrValid : Inport  Port=2
  startIn : Inport  Port=3
  dataIn : Inport  Port=4
  validIn : Inport  Port=5
  rstIn : Inport  Port=6
  maxPeakSearcher : Subsystem
  peakDetector : Subsystem
  lstfStart : Outport
  validOut : Outport  Port=2
  dataOut : Outport  Port=3
  wires:
  validIn/1 -> maxPeakSearcher/4(validIn)
  corrIn/1 -> maxPeakSearcher/1(corrIn)
  corrValid/1 -> maxPeakSearcher/2(corrValid)
  startIn/1 -> maxPeakSearcher/3(startIn)
  dataIn/1 -> maxPeakSearcher/5(dataIn)
  maxPeakSearcher/1(maxPeakValue) -> peakDetector/1(maxPeakVal)
  maxPeakSearcher/2(countRst) -> peakDetector/2(counterRst)
  maxPeakSearcher/3(dataOut) -> peakDetector/3(dataIn)
  maxPeakSearcher/4(validOut) -> peakDetector/4(validIn)
  peakDetector/1(lstfStart) -> lstfStart/1
  peakDetector/2(validOut) -> validOut/1
  peakDetector/3(dataOut) -> dataOut/1
  rstIn/1 -> maxPeakSearcher/6(rstIn)

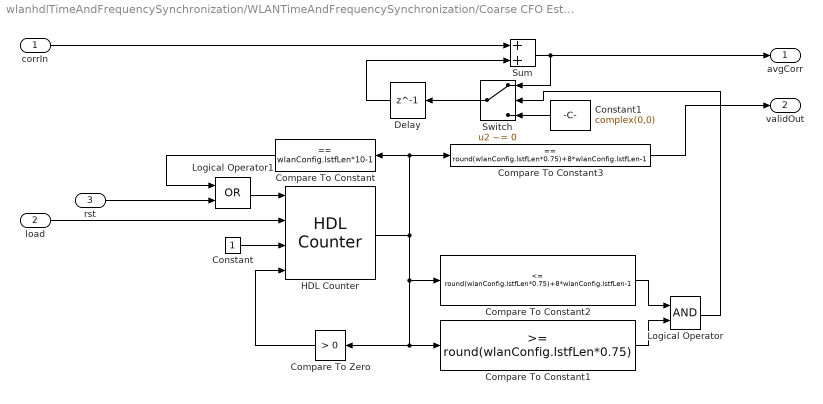
== system wlanhdlTimeAndFrequencySynchronization/WLANTimeAndFrequencySynchronization/Coarse CFO Estimation and Correction/Coarse CFO Estimation/Averager ==
  corrIn : Inport
  load : Inport  Port=2
  rst : Inport  Port=3
  Compare To Constant : simulink/Logic and Bit Operations/Compare To Constant  relop===  const=wlanConfig.lstfLen*10-1  OutDataTypeStr=boolean
      link override Compare: Operator===  OutDataTypeStr=boolean
  Compare To Constant1 : simulink/Logic and Bit Operations/Compare To Constant  relop=>=  const=round(wlanConfig.lstfLen*0.75)  OutDataTypeStr=boolean
      link override Compare: Operator=>=  OutDataTypeStr=boolean
  Compare To Constant2 : simulink/Logic and Bit Operations/Compare To Constant  relop=<=  const=round(wlanConfig.lstfLen*0.75)+8*wlanConfig.lstfLen-1  OutDataTypeStr=boolean
      link override Compare: Operator=<=  OutDataTypeStr=boolean
  Compare To Constant3 : simulink/Logic and Bit Operations/Compare To Constant  relop===  const=round(wlanConfig.lstfLen*0.75)+8*wlanConfig.lstfLen-1  OutDataTypeStr=boolean
      link override Compare: Operator===  OutDataTypeStr=boolean
  Compare To Zero : simulink/Logic and Bit Operations/Compare To Zero  relop=>  OutDataTypeStr=boolean
      link override Compare: Operator=>  OutDataTypeStr=boolean
  Constant : Constant  OutDataTypeStr=uint16  SampleTime=-1
  Constant1 : Constant  Value=complex(0,0)  OutDataTypeStr=Inherit: Inherit via back propagation  SampleTime=-1
  Delay : Delay  DelayLength=1
  HDL Counter : hdlsllib/Sources/HDL Counter  CountType=Count limited  CountInit=0  CountStep=1  CountMax=10*wlanConfig.lstfLen-1  CountFromType=Initial value  CountFrom=0  CountResetPort=on  CountLoadPort=on  CountEnbPort=on  CountDirPort=off  CountHitOutputPort=off  CountDataType=Unsigned  CountWordLen=16  CountFracLen=0  CountSampTime=1
      link override Add_wrap/Compare To Constant/Compare: Operator=>  OutDataTypeStr=boolean
      link override Sub_wrap/Compare To Constant/Compare: Operator=<  OutDataTypeStr=boolean
  Logical Operator : Logic  AllPortsSameDT=off  OutDataTypeStr=boolean
  Logical Operator1 : Logic  Operator=OR  AllPortsSameDT=off  OutDataTypeStr=boolean
  Sum : Sum  OutDataTypeStr=Inherit: Same as first input
  Switch : Switch  Criteria=u2 ~= 0  Threshold=1  SaturateOnIntegerOverflow=off  InputSameDT=off
  avgCorr : Outport
  validOut : Outport  Port=2
  wires:
  HDL Counter/1 -> Compare To Constant2/1, Compare To Constant1/1, Compare To Zero/1, Compare To Constant/1, Compare To Constant3/1
  Compare To Constant2/1 -> Logical Operator/1
  Constant/1 -> HDL Counter/3
  Sum/1 -> avgCorr/1, Switch/1
  Constant1/1 -> Switch/3
  corrIn/1 -> Sum/1
  Compare To Zero/1 -> HDL Counter/4
  Logical Operator1/1 -> HDL Counter/1
  Compare To Constant1/1 -> Logical Operator/2
  Logical Operator/1 -> Switch/2
  Compare To Constant/1 -> Logical Operator1/1
  Delay/1 -> Sum/2
  Switch/1 -> Delay/1
  rst/1 -> Logical Operator1/2
  Compare To Constant3/1 -> validOut/1
  load/1 -> HDL Counter/2

== system wlanhdlTimeAndFrequencySynchronization/WLANTimeAndFrequencySynchronization/Coarse CFO Estimation and Correction/Coarse CFO Estimation/Correlator ==
  dataIn : Inport
  lstf_start : Inport  Port=2
  Data Type Conversion : DataTypeConversion  OutDataTypeStr=fixdt(1,31,19)  SaturateOnIntegerOverflow=off  RndMeth=Floor
  Delay1 : Delay  InitialCondition=0  UseCircularBuffer=on
  Delay2 : Delay  DelayLength=wlanConfig.lstfLen  InitialCondition=0
  Delay3 : Delay  InitialCondition=0  UseCircularBuffer=on
  Delay4 : Delay  DelayLength=wlanConfig.lstfLen  InitialCondition=0
  Delay5 : Delay  InitialCondition=0  UseCircularBuffer=on
  Product : Product  RndMeth=Round
  complexConj : Math  Operator=conj  SignedPower=on  SaturateOnIntegerOverflow=off
  corrOut : Outport
  load : Outport  Port=2
  wires:
  dataIn/1 -> Delay2/1, Delay1/1
  Delay1/1 -> Product/1
  Product/1 -> Data Type Conversion/1
  Delay2/1 -> complexConj/1
  Delay3/1 -> Product/2
  complexConj/1 -> Delay3/1
  Data Type Conversion/1 -> corrOut/1
  lstf_start/1 -> Delay4/1
  Delay4/1 -> Delay5/1
  Delay5/1 -> load/1

== system wlanhdlTimeAndFrequencySynchronization/WLANTimeAndFrequencySynchronization/Coarse Time Sync/Correlator/MagnitudeSquared ==
  dataIn : Inport
  validIn : Inport  Port=2
  Add : Sum  OutDataTypeStr=Inherit: Same as accumulator
  Complex to Real-Imag : ComplexToRealImag
  Delay{,1..3} (4 alike) : Delay
  Delay4 : Delay  DelayLength=1
  Delay5 : Delay  DelayLength=1
  Delay6 : Delay  DelayLength=3
  Product1 : Product
  Product4 : Product
  dataOut : Outport  VectorParamsAs1DForOutWhenUnconnected=off
  validOut : Outport  Port=2  VectorParamsAs1DForOutWhenUnconnected=off
  wires:
  Complex to Real-Imag/2 -> Delay3/1, Delay2/1
  dataIn/1 -> Complex to Real-Imag/1
  validIn/1 -> Delay6/1
  Complex to Real-Imag/1 -> Delay1/1, Delay/1
  Product4/1 -> Delay4/1
  Product1/1 -> Delay5/1
  Add/1 -> dataOut/1
  Delay/1 -> Product4/2
  Delay1/1 -> Product4/1
  Delay2/1 -> Product1/1
  Delay3/1 -> Product1/2
  Delay4/1 -> Add/1
  Delay5/1 -> Add/2
  Delay6/1 -> validOut/1

== system wlanhdlTimeAndFrequencySynchronization/WLANTimeAndFrequencySynchronization/Coarse Time Sync/Correlator/MovingSum ==
  dataIn : Inport
  validIn : Inport  Port=2
  reset : Inport  Port=3
  Add : Sum  Inputs=|+-  OutDataTypeStr=Inherit: Same as accumulator
  Add1 : Sum  OutDataTypeStr=Inherit: Same as first input
  Delay{3..6,12} (5 alike) : Delay  DelayLength=1  InitialCondition=0
  Shift Arithmetic : ArithShift  BitShiftNumber=1  BitShiftDirection=Right
  "Synchronous Enabled 128 Sample Delay " : Subsystem
  Synchronous Enabled Unit Delay : hdlsllib/Discrete/Unit Delay Enabled Synchronous  InitialCondition=0.0  SampleTime=-1
  dataOut : Outport  VectorParamsAs1DForOutWhenUnconnected=off
  validOut : Outport  Port=2  VectorParamsAs1DForOutWhenUnconnected=off
  wires:
  "Synchronous Enabled 128 Sample Delay "/1(dataOut) -> Add/2
  Synchronous Enabled Unit Delay/1 -> Add1/1, Delay5/1
  dataIn/1 -> "Synchronous Enabled 128 Sample Delay "/1(dataIn), Add/1
  Delay6/1 -> validOut/1
  Delay5/1 -> dataOut/1
  Delay4/1 -> Delay6/1
  Delay3/1 -> Synchronous Enabled Unit Delay/2, Delay4/1
  validIn/1 -> Delay3/1, "Synchronous Enabled 128 Sample Delay "/2(en)
  Add/1 -> Shift Arithmetic/1
  Add1/1 -> Synchronous Enabled Unit Delay/1
  reset/1 -> "Synchronous Enabled 128 Sample Delay "/3(reset)
  Delay12/1 -> Add1/2
  Shift Arithmetic/1 -> Delay12/1

== system wlanhdlTimeAndFrequencySynchronization/WLANTimeAndFrequencySynchronization/Coarse Time Sync/Correlator/delayedCorrelation ==
  dataIn : Inport
  validIn : Inport  Port=2
  startIn : Inport  Port=3
  Conjugate : Math  Operator=conj  SignedPower=on  RndMeth=Zero
  DTadjust : MATLAB Function  TreatAsAtomicUnit=on
  Delay1 : Delay  DelayLength=wlanConfig.lstfLen
  Delay16 : Delay  DelayLength=wlanConfig.lstfLen
  Delay4 : Delay
  Delay5 : Delay
  Delay6 : Delay  DelayLength=1
  Delay7 : Delay  DelayLength=3
  Delay8 : Delay  DelayLength=3
  Product : Product
  corrOut : Outport
  corrValid : Outport  Port=2
  startOut : Outport  Port=3
  wires:
  dataIn/1 -> Delay4/1, Delay16/1
  Delay16/1 -> Conjugate/1
  Delay4/1 -> Product/1
  Conjugate/1 -> Delay5/1
  Delay5/1 -> Product/2
  startIn/1 -> Delay8/1
  Delay1/1 -> Delay7/1
  Product/1 -> Delay6/1
  validIn/1 -> Delay1/1
  Delay8/1 -> startOut/1
  Delay7/1 -> corrValid/1
  Delay6/1 -> DTadjust/1(in)
  DTadjust/1(out) -> corrOut/1

== system wlanhdlTimeAndFrequencySynchronization/WLANTimeAndFrequencySynchronization/Coarse Time Sync/Energy Calculator/magnitudeSquared ==
  dataIn : Inport
  validIn : Inport  Port=2
  Add : Sum
  Delay : Delay  DelayLength=wlanConfig.lstfLen
  Delay1 : Delay  DelayLength=wlanConfig.lstfLen
  Delay2 : Delay  DelayLength=wlanConfig.lstfLen-1
  Delay3 : Delay  DelayLength=1
  Delay4 : Delay  DelayLength=1
  MagnitudeSquared : Subsystem
  MagnitudeSquared1 : Subsystem
  MovingSum : Subsystem  InitFcn=Simulink.suppressDiagnostic(gcb, 'SimulinkFixedPoint:util:Overflowoccurred');
  Shift Arithmetic : ArithShift  BitShiftNumber=1  BitShiftDirection=Right
  Shift Arithmetic1 : ArithShift  BitShiftNumber=log2(wlanConfig.lstfLen)  BitShiftDirection=Right
  Shift Arithmetic2 : ArithShift  BitShiftNumber=1  BitShiftDirection=Right
  energy : Outport
  push : Outport  Port=2
  wires:
  validIn/1 -> MagnitudeSquared/2(validIn)
  dataIn/1 -> MagnitudeSquared/1(dataIn)
  MagnitudeSquared/1(dataOut) -> Delay3/1
  Delay/1 -> Add/2
  Add/1 -> Shift Arithmetic/1
  Shift Arithmetic/1 -> MovingSum/1(dataIn)
  MovingSum/1(dataOut) -> Shift Arithmetic1/1
  Shift Arithmetic1/1 -> MagnitudeSquared1/1(dataIn)
  Delay2/1 -> MagnitudeSquared1/2(validIn)
  MagnitudeSquared1/1(dataOut) -> Shift Arithmetic2/1
  MagnitudeSquared1/2(validOut) -> push/1
  Shift Arithmetic2/1 -> energy/1
  Delay1/1 -> MovingSum/2(validIn)
  Delay3/1 -> Delay/1, Add/1
  Delay4/1 -> Delay1/1
  MagnitudeSquared/2(validOut) -> Delay4/1
  MovingSum/2(validOut) -> Delay2/1

== system wlanhdlTimeAndFrequencySynchronization/WLANTimeAndFrequencySynchronization/Coarse Time Sync/Energy Calculator/streamSynchronizer ==
  corrValid : Inport
  energy : Inport  Port=2
  dataValid : Inport  Port=3
  Delay{1..4,6} (5 alike) : Delay  DelayLength=1
  StreamSyncronizer : MATLAB Function  InitFcn=Simulink.suppressDiagnostic(gcb, 'Stateflow:Runtime:DataOverflowErrorMSLD');  TreatAsAtomicUnit=on  mask{depth=256}
      mask help: Synchronize two data streams with a FIFO.
  dataOut : Outport
  validOut : Outport  Port=2
  wires:
  corrValid/1 -> Delay4/1
  Delay6/1 -> StreamSyncronizer/3(push)
  dataValid/1 -> Delay6/1
  Delay4/1 -> StreamSyncronizer/1(pop)
  energy/1 -> Delay1/1
  StreamSyncronizer/2(validOut) -> Delay3/1
  StreamSyncronizer/1(dataOut) -> Delay2/1
  Delay1/1 -> StreamSyncronizer/2(dataIn)
  Delay2/1 -> dataOut/1
  Delay3/1 -> validOut/1

== system wlanhdlTimeAndFrequencySynchronization/WLANTimeAndFrequencySynchronization/Coarse Time Sync/Peak Detector/considerFirstPeak ==
  peakIn : Inport
  Compare To Constant : simulink/Logic and Bit Operations/Compare To Constant  relop===  const=wlanConfig.lstfLen*10-1  OutDataTypeStr=boolean
      link override Compare: Operator===  OutDataTypeStr=boolean
  Compare To Constant1 : simulink/Logic and Bit Operations/Compare To Constant  relop===  const=0  OutDataTypeStr=boolean
      link override Compare: Operator===  OutDataTypeStr=boolean
  Delay{7,9..11} (4 alike) : Delay  DelayLength=1
  HDL Counter1 : hdlsllib/Sources/HDL Counter  CountType=Count limited  CountInit=0  CountStep=1  CountMax=wlanConfig.lstfLen*10-1  CountFromType=Initial value  CountFrom=0  CountResetPort=on  CountLoadPort=off  CountEnbPort=on  CountDirPort=off  CountHitOutputPort=off  CountDataType=Unsigned  CountWordLen=16  CountFracLen=0  CountSampTime=1
      link override Add_wrap/Compare To Constant/Compare: Operator=>  OutDataTypeStr=boolean
      link override Sub_wrap/Compare To Constant/Compare: Operator=<  OutDataTypeStr=boolean
  Logical Operator1 : Logic  AllPortsSameDT=off  OutDataTypeStr=boolean
  Logical Operator2 : Logic  Operator=OR  AllPortsSameDT=off  OutDataTypeStr=boolean
  Logical Operator6 : Logic  Operator=OR  AllPortsSameDT=off  OutDataTypeStr=boolean
  Logical Operator7 : Logic  AllPortsSameDT=off  OutDataTypeStr=boolean
  Switch : Switch  Criteria=u2 ~= 0  SaturateOnIntegerOverflow=off  InputSameDT=off
  peakOut : Outport
  validOut : Outport  Port=2
  wires:
  Logical Operator6/1 -> Delay10/1, Delay9/1
  HDL Counter1/1 -> Compare To Constant/1, Compare To Constant1/1
  Logical Operator2/1 -> Delay7/1, validOut/1
  Logical Operator1/1 -> Logical Operator7/2, Switch/3, Logical Operator6/1, Logical Operator2/1
  Delay10/1 -> Switch/2, Logical Operator7/1
  Compare To Constant/1 -> HDL Counter1/1
  peakIn/1 -> Logical Operator1/2, HDL Counter1/2
  Delay7/1 -> Logical Operator2/2
  Delay9/1 -> Logical Operator6/2
  Delay11/1 -> Switch/1
  Compare To Constant1/1 -> Logical Operator1/1
  Switch/1 -> peakOut/1
  Logical Operator7/1 -> Delay11/1
